simulink model "ex3_1"  (Simulink 7.4)
settings: Solver=FixedStepDiscrete  SolverMode=SingleTasking  StartTime=0.0  StopTime=inf  FixedStep=0.005  RelTol=1e-3
InitFcn:
  | Ts = 0.1;
  | disp(['Setting sample time to ' num2str(Ts) ' seconds'])
  | disp('To change this, go to: File -> Model Properties -> Callbacks')
  | disp('and change the Model initialization function')
libraries: dspsigops x20, dsparch4 x1
settings Model: Creator=fwornle  LastModifiedBy=fw  SimulationMode=external
settings ConfigSet: Description=rtmc9s12target_R2009b
settings DataIOCC: SignalLoggingName=sigsOut
settings OptimizationCC: InitFltsAndDblsToZero=on  OptimizeModelRefInitCode=on  LifeSpan=1
settings DebuggingCC: SaveWithParameterizedLinksMsg=none  SignalResolutionControl=TryResolveAllWithWarning  SolverPrmCheckMsg=none  MultiTaskDSMMsg=warning  MultiTaskCondExecSysMsg=none  StrictBusMsg=None
settings HardwareCC: ProdBitPerInt=16  ProdEndianess=BigEndian  ProdWordSize=16  ProdHWDeviceType=Motorola HC12
settings RTWCC: SystemTargetFile=mc9s12.tlc  GenerateMakefile=off  TemplateMakefile=mc9s12.tmf  ProcessScript=mc9s12_make_rtw_hook  IncludeERTFirstTime=on
settings STFCustomTargetCC: TargetFcnLib=ansi_tfl_tmw.mat  ModelReferenceCompliant=off  IncludeMdlTerminateFcn=off  ERTCustomFileBanners=on  SupportNonInlinedSFcns=off  CPPClassGenCompliant=on  SystemTargetFile=mc9s12.tlc
settings ERTTargetCC: TargetFcnLib=ansi_tfl_tmw.mat  MultiwordLength=2048  ModelReferenceCompliant=off  ParMdlRefBuildCompliant=off  CompOptLevelCompliant=off  IncludeMdlTerminateFcn=off  CombineOutputUpdateFcns=off  ERTFirstTimeCompliant=off  SupportContinuousTime=on  ModelStepFunctionPrototypeControlCompliant=off  ExtMode=on  ExtModeMexFile=ext_serial_mc9s12_comm  ExtModeMexArgs=1,2,115200  InlinedParameterPlacement=NonHierarchical  ERTCustomFileTemplate=mc9s12_file_process.tlc  GRTInterface=on  ConvertIfToSwitch=off
settings CustomProperty: DataType=RTWOptions_EnumType_C__Users_fw__SVN_rtmc9s12-target_trunk_rtmc9s12_CW_R2009b_bin_mc9s12_1mc9s12_TargetBoard  Value=Dragon12Plus
settings EnumStrPairs: String=Dragon12

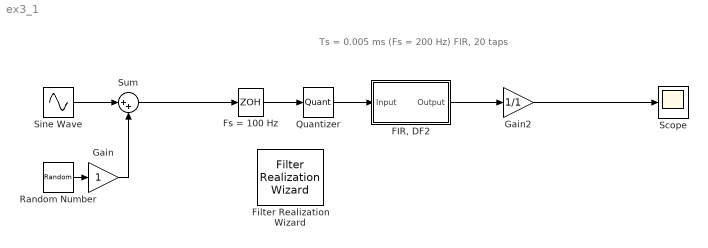
== system ex3_1 ==
  note: Ts = 0.005 ms
      | (Fs = 200 Hz)
      | FIR, 20 taps
  "FIR, DF2" : Subsystem  Tag=FilterWizardSubSystem
  Filter Realization Wizard : dsparch4/Filter Realization Wizard  SystemSampleTime=-1
  Fs = 100 Hz : ZeroOrderHold  SampleTime=0.01
  Gain : Gain  ParameterDataType=sfix(16)  ParameterScaling=2^0  OutDataType=sfix(16)  OutScaling=2^0  SaturateOnIntegerOverflow=on  OutDataTypeStr=Inherit: Same as input  ParamDataTypeStr=Inherit: Same as input
  Gain2 : Gain  Gain=1/1  ParameterDataType=sfix(16)  ParameterScaling=2^0  OutDataType=sfix(16)  OutScaling=2^0  SaturateOnIntegerOverflow=on  OutDataTypeStr=Inherit: Same as input  ParamDataTypeStr=Inherit: Same as input
  Quantizer : Quantizer  QuantizationInterval=2/(2^6-1)  LinearizeAsGain=off
  Random Number : RandomNumber  Variance=1e-6  SampleTime=0
  Scope : Scope
      settings: TimeRange=1  YMin=-1.5  YMax=1.5  SaveName=y1
  Sine Wave : Sin  Amplitude=1  Bias=0  Frequency=2*pi*20  Phase=0  Samples=10  SampleTime=0  Offset=0
  Sum : Sum  Inputs=|++  OutDataType=sfix(16)  OutScaling=2^0  SaturateOnIntegerOverflow=on
  wires:
  Random Number/1 -> Gain/1
  Gain/1 -> Sum/2
  Fs = 100 Hz/1 -> Quantizer/1
  Sine Wave/1 -> Sum/1
  "FIR, DF2"/1(Output) -> Gain2/1
  Sum/1 -> Fs = 100 Hz/1
  Quantizer/1 -> "FIR, DF2"/1(Input)
  Gain2/1 -> Scope/1

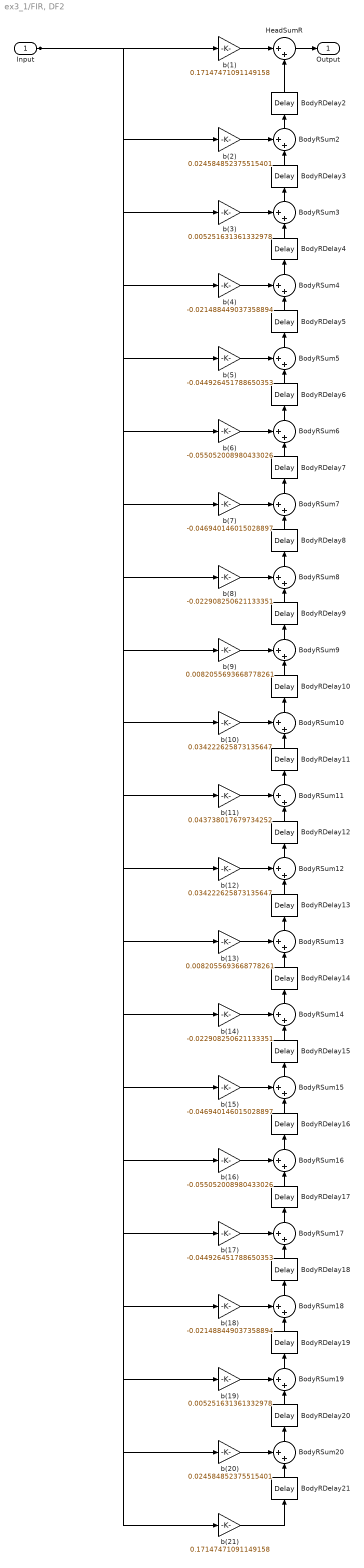
== system ex3_1/FIR, DF2 ==
  Input : Inport  OutDataType=sfix(16)  OutScaling=2^0
  BodyRDelay{2..21} (20 alike) : dspsigops/Delay  dly_unit=Samples  delay=1  ic_detail=off  dif_ic_for_ch=off  dif_ic_for_dly=off  ic=0  reset_popup=None
  BodyRSum{2..20} (19 alike) : Sum  Inputs=++|  OutDataType=sfix(16)  OutScaling=2^0  SaturateOnIntegerOverflow=on  InputSameDT=on  OutDataTypeStr=Inherit: Same as first input
  HeadSumR : Sum  Inputs=|++  OutDataType=sfix(16)  OutScaling=2^0  SaturateOnIntegerOverflow=on  InputSameDT=on  OutDataTypeStr=Inherit: Same as first input
  b(1) : Gain  Gain=0.17147471091149158  ParameterDataType=sfix(16)  ParameterScaling=2^0  OutDataType=sfix(16)  OutScaling=2^0  SaturateOnIntegerOverflow=on  OutDataTypeStr=Inherit: Same as input  ParamDataTypeStr=Inherit: Same as input
  b(10) : Gain  Gain=0.034222625873135647  ParameterDataType=sfix(16)  ParameterScaling=2^0  OutDataType=sfix(16)  OutScaling=2^0  SaturateOnIntegerOverflow=on  OutDataTypeStr=Inherit: Same as input  ParamDataTypeStr=Inherit: Same as input
  b(11) : Gain  Gain=0.043738017679734252  ParameterDataType=sfix(16)  ParameterScaling=2^0  OutDataType=sfix(16)  OutScaling=2^0  SaturateOnIntegerOverflow=on  OutDataTypeStr=Inherit: Same as input  ParamDataTypeStr=Inherit: Same as input
  b(12) : Gain  Gain=0.034222625873135647  ParameterDataType=sfix(16)  ParameterScaling=2^0  OutDataType=sfix(16)  OutScaling=2^0  SaturateOnIntegerOverflow=on  OutDataTypeStr=Inherit: Same as input  ParamDataTypeStr=Inherit: Same as input
  b(13) : Gain  Gain=0.0082055693668778261  ParameterDataType=sfix(16)  ParameterScaling=2^0  OutDataType=sfix(16)  OutScaling=2^0  SaturateOnIntegerOverflow=on  OutDataTypeStr=Inherit: Same as input  ParamDataTypeStr=Inherit: Same as input
  b(14) : Gain  Gain=-0.022908250621133351  ParameterDataType=sfix(16)  ParameterScaling=2^0  OutDataType=sfix(16)  OutScaling=2^0  SaturateOnIntegerOverflow=on  OutDataTypeStr=Inherit: Same as input  ParamDataTypeStr=Inherit: Same as input
  b(15) : Gain  Gain=-0.046940146015028897  ParameterDataType=sfix(16)  ParameterScaling=2^0  OutDataType=sfix(16)  OutScaling=2^0  SaturateOnIntegerOverflow=on  OutDataTypeStr=Inherit: Same as input  ParamDataTypeStr=Inherit: Same as input
  b(16) : Gain  Gain=-0.055052008980433026  ParameterDataType=sfix(16)  ParameterScaling=2^0  OutDataType=sfix(16)  OutScaling=2^0  SaturateOnIntegerOverflow=on  OutDataTypeStr=Inherit: Same as input  ParamDataTypeStr=Inherit: Same as input
  b(17) : Gain  Gain=-0.044926451788650353  ParameterDataType=sfix(16)  ParameterScaling=2^0  OutDataType=sfix(16)  OutScaling=2^0  SaturateOnIntegerOverflow=on  OutDataTypeStr=Inherit: Same as input  ParamDataTypeStr=Inherit: Same as input
  b(18) : Gain  Gain=-0.021488449037358894  ParameterDataType=sfix(16)  ParameterScaling=2^0  OutDataType=sfix(16)  OutScaling=2^0  SaturateOnIntegerOverflow=on  OutDataTypeStr=Inherit: Same as input  ParamDataTypeStr=Inherit: Same as input
  b(19) : Gain  Gain=0.005251631361332978  ParameterDataType=sfix(16)  ParameterScaling=2^0  OutDataType=sfix(16)  OutScaling=2^0  SaturateOnIntegerOverflow=on  OutDataTypeStr=Inherit: Same as input  ParamDataTypeStr=Inherit: Same as input
  b(2) : Gain  Gain=0.024584852375515401  ParameterDataType=sfix(16)  ParameterScaling=2^0  OutDataType=sfix(16)  OutScaling=2^0  SaturateOnIntegerOverflow=on  OutDataTypeStr=Inherit: Same as input  ParamDataTypeStr=Inherit: Same as input
  b(20) : Gain  Gain=0.024584852375515401  ParameterDataType=sfix(16)  ParameterScaling=2^0  OutDataType=sfix(16)  OutScaling=2^0  SaturateOnIntegerOverflow=on  OutDataTypeStr=Inherit: Same as input  ParamDataTypeStr=Inherit: Same as input
  b(21) : Gain  Gain=0.17147471091149158  ParameterDataType=sfix(16)  ParameterScaling=2^0  OutDataType=sfix(16)  OutScaling=2^0  SaturateOnIntegerOverflow=on  OutDataTypeStr=Inherit: Same as input  ParamDataTypeStr=Inherit: Same as input
  b(3) : Gain  Gain=0.005251631361332978  ParameterDataType=sfix(16)  ParameterScaling=2^0  OutDataType=sfix(16)  OutScaling=2^0  SaturateOnIntegerOverflow=on  OutDataTypeStr=Inherit: Same as input  ParamDataTypeStr=Inherit: Same as input
  b(4) : Gain  Gain=-0.021488449037358894  ParameterDataType=sfix(16)  ParameterScaling=2^0  OutDataType=sfix(16)  OutScaling=2^0  SaturateOnIntegerOverflow=on  OutDataTypeStr=Inherit: Same as input  ParamDataTypeStr=Inherit: Same as input
  b(5) : Gain  Gain=-0.044926451788650353  ParameterDataType=sfix(16)  ParameterScaling=2^0  OutDataType=sfix(16)  OutScaling=2^0  SaturateOnIntegerOverflow=on  OutDataTypeStr=Inherit: Same as input  ParamDataTypeStr=Inherit: Same as input
  b(6) : Gain  Gain=-0.055052008980433026  ParameterDataType=sfix(16)  ParameterScaling=2^0  OutDataType=sfix(16)  OutScaling=2^0  SaturateOnIntegerOverflow=on  OutDataTypeStr=Inherit: Same as input  ParamDataTypeStr=Inherit: Same as input
  b(7) : Gain  Gain=-0.046940146015028897  ParameterDataType=sfix(16)  ParameterScaling=2^0  OutDataType=sfix(16)  OutScaling=2^0  SaturateOnIntegerOverflow=on  OutDataTypeStr=Inherit: Same as input  ParamDataTypeStr=Inherit: Same as input
  b(8) : Gain  Gain=-0.022908250621133351  ParameterDataType=sfix(16)  ParameterScaling=2^0  OutDataType=sfix(16)  OutScaling=2^0  SaturateOnIntegerOverflow=on  OutDataTypeStr=Inherit: Same as input  ParamDataTypeStr=Inherit: Same as input
  b(9) : Gain  Gain=0.0082055693668778261  ParameterDataType=sfix(16)  ParameterScaling=2^0  OutDataType=sfix(16)  OutScaling=2^0  SaturateOnIntegerOverflow=on  OutDataTypeStr=Inherit: Same as input  ParamDataTypeStr=Inherit: Same as input
  Output : Outport  OutDataType=sfix(16)  OutScaling=2^0
  wires:
  Input/1 -> b(1)/1, b(2)/1, b(3)/1, b(4)/1, b(5)/1, b(6)/1, b(7)/1, b(8)/1, b(9)/1, b(10)/1, b(11)/1, b(12)/1, b(13)/1, b(14)/1, b(15)/1, b(16)/1, b(17)/1, b(18)/1, b(19)/1, b(20)/1, b(21)/1
  b(1)/1 -> HeadSumR/1
  HeadSumR/1 -> Output/1
  b(2)/1 -> BodyRSum2/1
  BodyRSum2/1 -> BodyRDelay2/1
  BodyRDelay2/1 -> HeadSumR/2
  b(3)/1 -> BodyRSum3/1
  BodyRSum3/1 -> BodyRDelay3/1
  BodyRDelay3/1 -> BodyRSum2/2
  b(4)/1 -> BodyRSum4/1
  BodyRSum4/1 -> BodyRDelay4/1
  BodyRDelay4/1 -> BodyRSum3/2
  b(5)/1 -> BodyRSum5/1
  BodyRSum5/1 -> BodyRDelay5/1
  BodyRDelay5/1 -> BodyRSum4/2
  b(6)/1 -> BodyRSum6/1
  BodyRSum6/1 -> BodyRDelay6/1
  BodyRDelay6/1 -> BodyRSum5/2
  b(7)/1 -> BodyRSum7/1
  BodyRSum7/1 -> BodyRDelay7/1
  BodyRDelay7/1 -> BodyRSum6/2
  b(8)/1 -> BodyRSum8/1
  BodyRSum8/1 -> BodyRDelay8/1
  BodyRDelay8/1 -> BodyRSum7/2
  b(9)/1 -> BodyRSum9/1
  BodyRSum9/1 -> BodyRDelay9/1
  BodyRDelay9/1 -> BodyRSum8/2
  b(10)/1 -> BodyRSum10/1
  BodyRSum10/1 -> BodyRDelay10/1
  BodyRDelay10/1 -> BodyRSum9/2
  b(11)/1 -> BodyRSum11/1
  BodyRSum11/1 -> BodyRDelay11/1
  BodyRDelay11/1 -> BodyRSum10/2
  b(12)/1 -> BodyRSum12/1
  BodyRSum12/1 -> BodyRDelay12/1
  BodyRDelay12/1 -> BodyRSum11/2
  b(13)/1 -> BodyRSum13/1
  BodyRSum13/1 -> BodyRDelay13/1
  BodyRDelay13/1 -> BodyRSum12/2
  b(14)/1 -> BodyRSum14/1
  BodyRSum14/1 -> BodyRDelay14/1
  BodyRDelay14/1 -> BodyRSum13/2
  b(15)/1 -> BodyRSum15/1
  BodyRSum15/1 -> BodyRDelay15/1
  BodyRDelay15/1 -> BodyRSum14/2
  b(16)/1 -> BodyRSum16/1
  BodyRSum16/1 -> BodyRDelay16/1
  BodyRDelay16/1 -> BodyRSum15/2
  b(17)/1 -> BodyRSum17/1
  BodyRSum17/1 -> BodyRDelay17/1
  BodyRDelay17/1 -> BodyRSum16/2
  b(18)/1 -> BodyRSum18/1
  BodyRSum18/1 -> BodyRDelay18/1
  BodyRDelay18/1 -> BodyRSum17/2
  b(19)/1 -> BodyRSum19/1
  BodyRSum19/1 -> BodyRDelay19/1
  BodyRDelay19/1 -> BodyRSum18/2
  b(20)/1 -> BodyRSum20/1
  BodyRSum20/1 -> BodyRDelay20/1
  BodyRDelay20/1 -> BodyRSum19/2
  b(21)/1 -> BodyRDelay21/1
  BodyRDelay21/1 -> BodyRSum20/2
